simulink model "day01"  (R2026a)
settings: Solver=VariableStepAuto  StopTime=inf
libraries: simulink x4
settings Model: Creator=pete  LastModifiedBy=pete

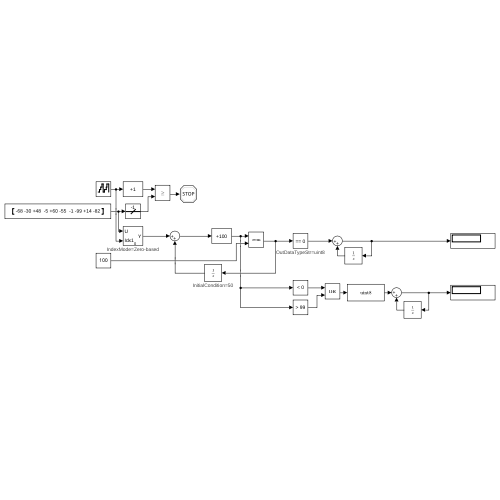
[thumbnail: Simulink's stored preview of the top-level diagram]
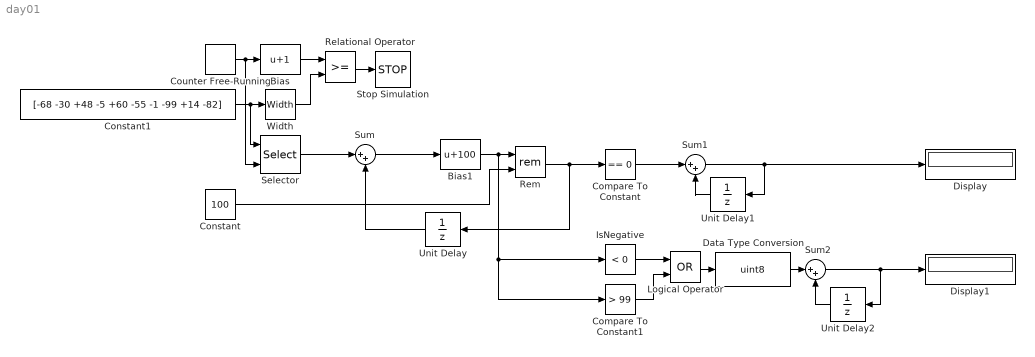
== system day01 ==
  Bias : Bias  Bias=1  SaturateOnIntegerOverflow=off
  Bias1 : Bias  Bias=100  SaturateOnIntegerOverflow=off
  Compare To Constant : simulink/Logic and Bit Operations/Compare To Constant  relop===  const=0  OutDataTypeStr=uint8
      settings: AttributesFormatString=OutDataTypeStr=%<OutDataTypeStr>
  Compare To Constant1 : simulink/Logic and Bit Operations/Compare To Constant  relop=>  const=99  OutDataTypeStr=boolean
  Constant : Constant  Value=100
  Constant1 : Constant  Value=[-68 -30 +48 -5 +60 -55 -1 -99 +14 -82]
  Counter Free-Running : simulink/Sources/Counter Free-Running  NumBits=16  tsamp=-1
  Data Type Conversion : DataTypeConversion  OutDataTypeStr=uint8  SaturateOnIntegerOverflow=off  RndMeth=Floor
  Display : Display
  Display1 : Display
  IsNegative : simulink/Logic and Bit Operations/Compare To Zero  relop=<  OutDataTypeStr=boolean
      settings: LibrarySourceBlock=|
      | simulink/Quick Insert/Logic and Bit
      | Operations/IsNegative
  Logical Operator : Logic  Operator=OR  AllPortsSameDT=off  OutDataTypeStr=boolean
  Relational Operator : RelationalOperator  OutDataTypeStr=boolean  RndMeth=Simplest  InputSameDT=off
  Rem : Math  Operator=rem
  Selector : Selector  IndexMode=Zero-based  InputPortWidth=10  IndexOptions=Index vector (port)  Indices=[1 3]  OutputSizes=1
      settings: AttributesFormatString=IndexMode=%<IndexMode>
  Stop Simulation : Stop
  Sum : Sum  Inputs=|++
  Sum1 : Sum  Inputs=|++
  Sum2 : Sum  Inputs=|++
  Unit Delay : UnitDelay  InitialCondition=50  SampleTime=-1
      settings: AttributesFormatString=InitialCondition=%<InitialCondition>
  Unit Delay1 : UnitDelay  SampleTime=-1
  Unit Delay2 : UnitDelay  SampleTime=-1
  Width : Width
  wires:
  Counter Free-Running/1 -> Selector/2, Bias/1
  Bias/1 -> Relational Operator/1
  Relational Operator/1 -> Stop Simulation/1
  Width/1 -> Relational Operator/2
  Selector/1 -> Sum/1
  Sum/1 -> Bias1/1
  Bias1/1 -> Compare To Constant1/1, IsNegative/1, Rem/1
  Rem/1 -> Compare To Constant/1, Unit Delay/1
  Unit Delay/1 -> Sum/2
  Compare To Constant/1 -> Sum1/1
  Sum1/1 -> Display/1, Unit Delay1/1
  Unit Delay1/1 -> Sum1/2
  Constant/1 -> Rem/2
  Constant1/1 -> Selector/1, Width/1
  IsNegative/1 -> Logical Operator/1
  Compare To Constant1/1 -> Logical Operator/2
  Logical Operator/1 -> Data Type Conversion/1
  Data Type Conversion/1 -> Sum2/1
  Sum2/1 -> Display1/1, Unit Delay2/1
  Unit Delay2/1 -> Sum2/2
